simulink model "example_layerwall_dynamic_mdl"  (R2013b)
settings: Solver=ode45  StartTime=0.0  StopTime=2*365*24*3600  MaxStep=3600  RelTol=1e-3
libraries: carnot x2
settings Model: Creator=drhf  LastModifiedBy=drhf
settings OptimizationCC: InlineParams=on

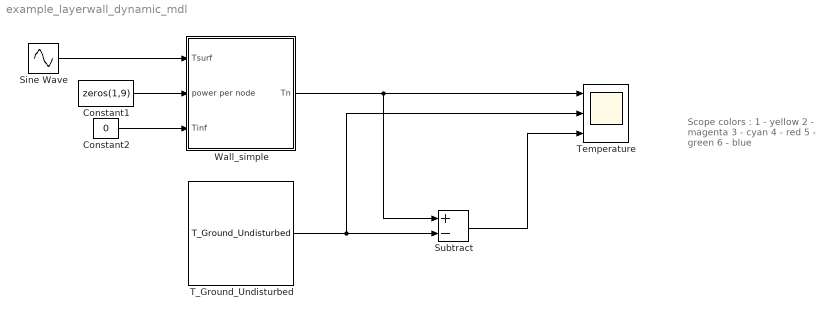
== system example_layerwall_dynamic_mdl ==
  note: Scope colors :
      | 1 - yellow
      | 2 - magenta
      | 3 - cyan
      | 4 - red
      | 5 - green
      | 6 - blue
  Constant1 : Constant  Value=zeros(1,9)
  Constant2 : Constant  Value=0
  Sine Wave : Sin  Amplitude=10  Frequency=2*pi/(3600*8760)  Phase=1.5*pi  SampleTime=0
  Subtract : Sum  Inputs=+-
  T_Ground_Undisturbed : carnot/Basic/Thermal_Models/T_Ground_Undisturbed  Tmeanoutside=11  deltathetae=9.3  tshift=319  cond_ground=2  rhocp=800*2500  hh=5  znodes=1
  Temperature : Scope  NumInputPorts=3
      settings: YMin=-5~-5~-5  YMax=5~5~5
  Wall_simple : Subsystem  mask(simplified wall){wallsize=[1 1], d=ones(1,10)*1, cond=ones(1,10)*1, cwall=ones(1,10)*1000, rho=ones(1,10)*2000, emission_in=.96, dactive=1:9, t0=0, tau=10000*3600}
      mask prompts: wallsize "size of wall [m] [height width]"; d "thickness of layers [m] (vector) (0 = towards this room)"; cond "conductivity of layers [W/(m*K)] (vector)"; cwall "capacity of layers [J/(kg*K)] (vector)"; rho "density of layers [kg/m³]"; emission_in "emission of wall surface"; dactive "depth active layer in m from inner surface  (-1 = none)"; t0 "initial temperature [degree centigrade]"; tau "time-constant of wall [s]"
      mask help: simplified model to test wall_basic
      mask init:
      | position = [0 90 0 ];
      | % nodes = length(d);
      | wallheight = wallsize(1);
      | wallsurface = wallsize(1)*wallsize(2);
      | 
      | if (dactive>=0) 
      |     active = 1;
      | else
      |     active = 0;
      | end
  wires:
  Sine Wave/1 -> Wall_simple/1(Tsurf)
  Wall_simple/1(Tn) -> Temperature/1, Subtract/1
  Constant1/1 -> Wall_simple/2(power per node)
  Constant2/1 -> Wall_simple/3(Tinf)
  T_Ground_Undisturbed/1 -> Temperature/2, Subtract/2
  Subtract/1 -> Temperature/3

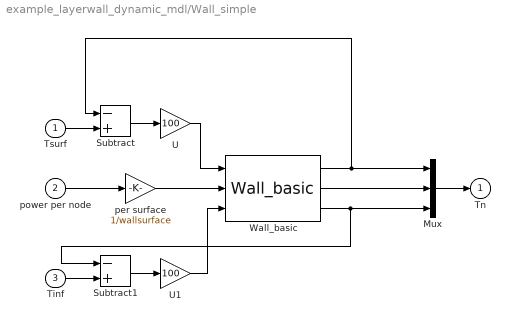
== system example_layerwall_dynamic_mdl/Wall_simple ==
  Tsurf : Inport
  power per node : Inport  Port=2
  Tinf : Inport  Port=3
  Mux : Mux  Inputs=3
  Subtract : Sum  Inputs=-+
  Subtract1 : Sum  Inputs=-+
  U : Gain  Gain=100  SaturateOnIntegerOverflow=on  OutDataTypeStr=Inherit: Same as input  ParamDataTypeStr=Inherit: Same as input
  U1 : Gain  Gain=100  SaturateOnIntegerOverflow=on  OutDataTypeStr=Inherit: Same as input  ParamDataTypeStr=Inherit: Same as input
  Wall_basic : carnot/Basic/Thermal_Models/Wall_basic  tau=tau  t0=t0  d=d  dactive=dactive  cond=cond  cwall=cwall  rho=rho
  per surface : Gain  Gain=1/wallsurface  SaturateOnIntegerOverflow=on  OutDataTypeStr=Inherit: Same as input  ParamDataTypeStr=Inherit: Same as input
  Tn : Outport
  wires:
  power per node/1 -> per surface/1
  per surface/1 -> Wall_basic/2
  Wall_basic/1 -> Subtract/1, Mux/1
  Wall_basic/3 -> Subtract1/1, Mux/3
  Wall_basic/2 -> Mux/2
  Mux/1 -> Tn/1
  Tsurf/1 -> Subtract/2
  Subtract/1 -> U/1
  U/1 -> Wall_basic/1
  Subtract1/1 -> U1/1
  Tinf/1 -> Subtract1/2
  U1/1 -> Wall_basic/3
